simulink model "bh_proto_swingup_OUT_OF_PHASE_CONTROL"  (R2017a)
settings: Solver=ode45  StartTime=0.0  StopTime=22  FixedStep=0.001  RelTol=1e-5  EnableMultiTasking=on
values from neighbouring files (symbols this model uses):
  b3_damp = res_T.b3_damp    [bh_pend_solve_ODE_sys.m]
  Io3_xx = res_T.Io3_xx    [bh_pend_solve_ODE_sys.m]
  L3y = res_T.L3y    [bh_pend_solve_ODE_sys.m]    (also in bh_pend_solve_ODE_sys_custom.m)
  m = res_T.mass3    [bh_pend_solve_ODE_sys_custom.m]
  mass3 = res_T.mass3    [bh_pend_solve_ODE_sys.m]    (also in bh_pend_solve_ODE_sys_custom.m)
  N = 1 + N_steps    [bh_pend_solve_ODE_sys_custom.m]
undefined symbols (not defined in the file or in its folder): L3x, L3z, X, Y, Z
libraries: sm_lib x12, simulink_extras x11, nesl_utility x8, simulink x1
settings Model: Creator=bhorton  LastModifiedBy=bhorton
settings SolverCC: ZeroCrossAlgorithm=Adaptive
settings OptimizationCC: LifeSpan=inf
settings DebuggingCC: SFUnexpectedBacktrackingDiag=warning  SFNoUnconditionalDefaultTransitionDiag=warning  SFExecutionAtInitializationDiag=none
settings GRTTargetCC: TargetLangStandard=C89/C90 (ANSI)
settings ConfigComp: CovMetricSettings=dw  CovHtmlReporting=on  CovSaveCumulativeToWorkspaceVar=on  CovSaveSingleToWorkspaceVar=on  CovExternalEMLEnable=off
settings SimscapeCC: SimscapeLogDataHistory=10000  SelectedTab=Simscape Multibody
settings ExplorerConfigSet: InternalSimMechanicsExplorerSettings="<ExplorerConfiguration><canonicalview>default</canonicalview><AnimationSetting><BasePlaybackSpeed>1.0</BasePlaybackSpeed><PlaybackSpeedFactor>1.0</PlaybackSpeedFactor></AnimationSetting><TilePanel><TileInfo><Tiles Columns=\"1\" Count=\"1\" Rows=\"1\"><Column Left=\"2\" Weight=\"1\"/><Column Left=\"1585\" Weight=\"0.5\"/><Row Top=\"2\" Weight=\"1\"/><Row Top=\"911\" Weight=\"0.5005\"/><Tile Height=\"1\" Width=\"1\" X=\"0\" Y=\"0\"/></Tiles></TileInfo><SceneInfo><SceneViewer><BGColor><R>0.60000002384185791</R><G>0.60000002384185791</G><B>0.60000002384185791</B></BGColor><Camera><DoPerspective>off</DoPerspective><Position><X>0.97226610796774449</X><Y>0.24871023220719646</Y><Z>0.19848014681163439</Z></Position><Center><X>-1.1885447515069814e-08</X><Y>0.12499999495795672</Y><Z>-1.7810067587387124e-09</Z></Center><Up><X>-0.2183009159559649</X><Y>0.17550270816811642</Y><Z>0.9599705774233106</Z></Up><ViewLimDist>1</ViewLimDist><YLim>0.073618170266836078</YLim><XLim>0.12874999999999998</XLim></Camera></SceneViewer></SceneInfo></TilePanel><MechEditorPanel><Cameras/><GfxPanelCameraMap/><VideoCreator><PlaybackSpeedRatio>1.0</PlaybackSpeedRatio><FrameRate>30</FrameRate><VideoFormat>Motion JPEG AVI</VideoFormat><FrameSize>auto</FrameSize></VideoCreator></MechEditorPanel></ExplorerConfiguration>"

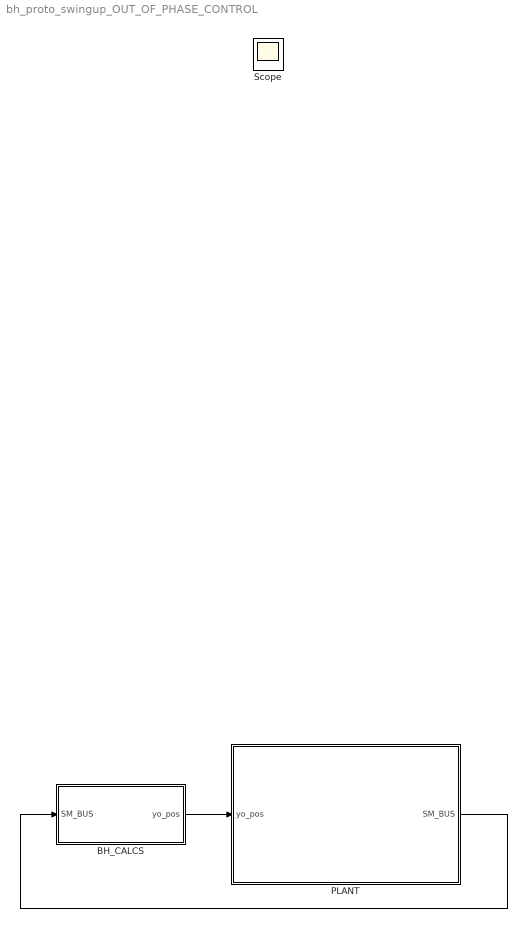
== system bh_proto_swingup_OUT_OF_PHASE_CONTROL ==
  BH_CALCS : Subsystem
  PLANT : Subsystem
  Scope : Scope
  wires:
  PLANT/1(SM_BUS) -> BH_CALCS/1(SM_BUS)
  BH_CALCS/1(yo_pos) -> PLANT/1(yo_pos)

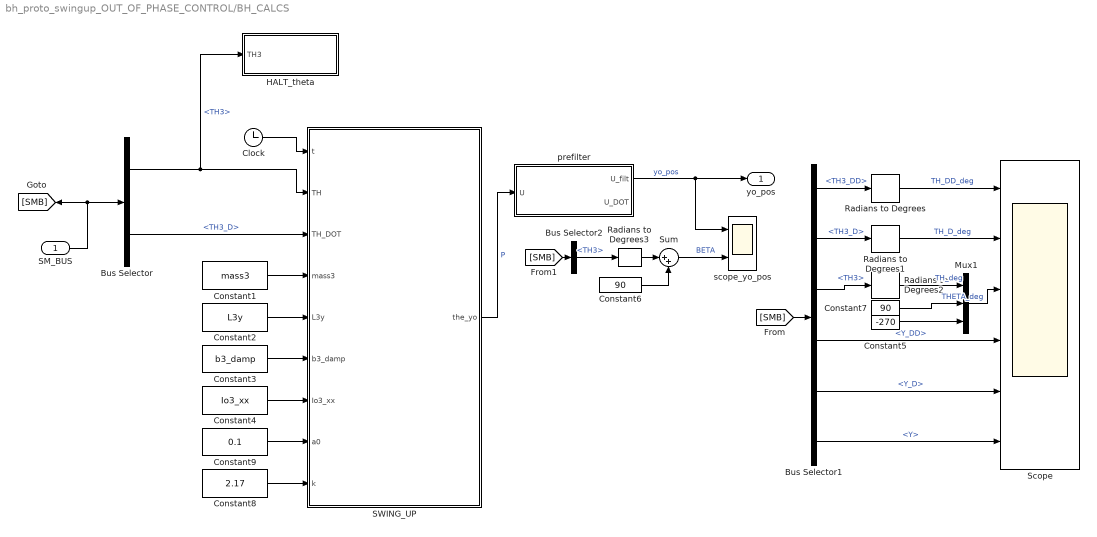
== system bh_proto_swingup_OUT_OF_PHASE_CONTROL/BH_CALCS ==
  SM_BUS : Inport
  Bus Selector : BusSelector  OutputSignals=TH3,TH3_D
  Bus Selector1 : BusSelector  OutputSignals=TH3_DD,TH3_D,TH3,Y_DD,Y_D,Y
  Bus Selector2 : BusSelector  OutputSignals=TH3
  Clock : Clock
  Constant1 : Constant  Value=mass3
  Constant2 : Constant  Value=L3y
  Constant3 : Constant  Value=b3_damp
  Constant4 : Constant  Value=Io3_xx
  Constant5 : Constant  Value=-270
  Constant6 : Constant  Value=90
  Constant7 : Constant  Value=90
  Constant8 : Constant  Value=2.17
  Constant9 : Constant  Value=0.1
  HALT_theta : Subsystem
  Mux1 : Mux  Inputs=3
  Radians to Degrees{,1..3} (4 alike) : simulink_extras/Transformations/Radians to Degrees
  SWING_UP : MATLAB Function  TreatAsAtomicUnit=on  SystemSampleTime=0.001
  Scope : Scope  NumInputPorts=6
  Sum : Sum  Inputs=|++
  prefilter : Subsystem  mask(Derivative Estimation){wn=2*pi*50, p=1}
      mask prompts: wn "Natural frequency, wn (rad/sec)"; p "Damping ratio, p"
      mask help:
      | A simple derivative estimator using a 2nd order representation between input and output.
      |
      | The integrators use a discrete FORWARd Euler rule, and a sample time needs to be specified.
      mask init:
      | str1 = sprintf('wn = %.2f', wn);
      | str2 = sprintf('p  = %.2f', p);
      | %str3 = sprintf('dt = %.2f', dt);
      | %str = char(str1,str2,str3);
      | %str3 = sprintf('dt = %.2f', dt);
      | str = char(str1,str2);
      mask Display: disp(str)
  scope_yo_pos : Scope  NumInputPorts=2
  yo_pos : Outport
  wires:
  prefilter/1(U_filt) -> scope_yo_pos/1, yo_pos/1  "yo_pos"
  SM_BUS/1 -> [SMB], Bus Selector/1
  Bus Selector/1 -> SWING_UP/2(TH), HALT_theta/1(TH3)  "<TH3>"
  Bus Selector/2 -> SWING_UP/3(TH_DOT)  "<TH3_D>"
  Constant3/1 -> SWING_UP/6(b3_damp)
  Constant2/1 -> SWING_UP/5(L3y)
  Constant1/1 -> SWING_UP/4(mass3)
  [SMB] -> Bus Selector1/1
  Bus Selector1/1 -> Radians to Degrees/1  "<TH3_DD>"
  Bus Selector1/2 -> Radians to Degrees1/1  "<TH3_D>"
  Bus Selector1/3 -> Radians to Degrees2/1  "<TH3>"
  Radians to Degrees/1 -> Scope/1  "TH_DD_deg"
  Radians to Degrees1/1 -> Scope/2  "TH_D_deg"
  Radians to Degrees2/1 -> Mux1/1  "TH_deg"
  Bus Selector1/4 -> Scope/4  "<Y_DD>"
  Bus Selector1/5 -> Scope/5  "<Y_D>"
  Bus Selector1/6 -> Scope/6  "<Y>"
  Clock/1 -> SWING_UP/1(t)
  Constant4/1 -> SWING_UP/7(Io3_xx)
  Constant7/1 -> Mux1/2
  Constant9/1 -> SWING_UP/8(a0)
  Constant8/1 -> SWING_UP/9(k)
  Mux1/1 -> Scope/3  "THETA_deg"
  Constant5/1 -> Mux1/3
  SWING_UP/1(the_yo) -> prefilter/1(U)  "P"
  [SMB] -> Bus Selector2/1
  Sum/1 -> scope_yo_pos/2  "BETA"
  Bus Selector2/1 -> Radians to Degrees3/1  "<TH3>"
  Radians to Degrees3/1 -> Sum/1
  Constant6/1 -> Sum/2

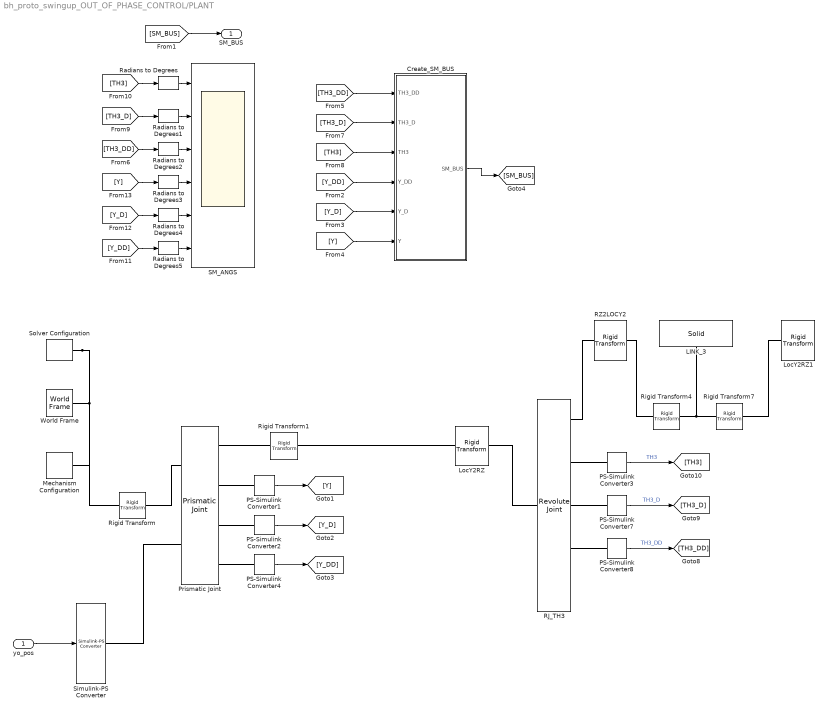
== system bh_proto_swingup_OUT_OF_PHASE_CONTROL/PLANT ==
  yo_pos : Inport
  Create_SM_BUS : Subsystem
  LINK_3 : sm_lib/Body Elements/Solid  InertiaType=CalculateFromGeometry  Mass=1  MassUnits=kg  CenterOfMass=[0 0 0]  CenterOfMassUnits=m  MomentsOfInertia=[1 1 1]  MomentsOfInertiaUnits=kg*m^2  ProductsOfInertia=[0 0 0]  ProductsOfInertiaUnits=kg*m^2  DensityBased=on  Density=density  DensityUnits=kg/(m^3)  DoExposeReferenceFrame=on  SerializedFrames=<Frames/>  GraphicType=FromGeometry  MarkerShape=Sphere  MarkerSize=10  GraphicVisPropType=SimpleVisualProperties  GraphicDiffuseColor=[1.0 0.8 0.4]  GraphicSpecularColor=[0.5 0.5 0.5 1.0]  GraphicAmbientColor=[0.15 0.15 0.15 1.0]  GraphicEmissiveColor=[0.0 0.0 0.0 1.0]  GraphicShininess=75  GraphicOpacity=1.0  GeometryShape=Brick  RectangleSize=[1 1]  RectangleSizeUnits=m  BrickDimensions=[L3x, L3y, L3z ]  BrickDimensionUnits=m  CylinderRadius=1  CylinderRadiusUnits=m  CylinderLength=1  CylinderLengthUnits=m  SphereRadius=1  SphereRadiusUnits=m  EllipsoidRadii=[1 1 1]  EllipsoidRadiiUnits=m  ExtrusionCrossSection=[1 1; -1 1; -1 -1; 1 -1]  ExtrusionCrossSectionUnits=m  ExtrusionLength=1  ExtrusionLengthUnits=m  PolygonNumSides=3  PolygonOuterRadius=1  PolygonOuterRadiusUnits=m  ExtGeomFileType=STEP  ExtGeomFileUnits=m  RevolutionCrossSection=[1 1; 1 -1; 2 -1; 2 1]  RevolutionCrossSectionUnits=m  RevolutionExtent=Full  RevolutionAngle=180  RevolutionAngleUnits=deg
  LocY2RZ : sm_lib/Frames and Transforms/Rigid Transform  TranslationMethod=None  TranslationStandardOffset=0  TranslationLengthUnit=m  TranslationStandardAxis=+Z  TranslationCartesianOffset=[0 0 0]  TranslationROffset=0  TranslationROffsetUnits=m  TranslationZOffset=0  TranslationZOffsetUnits=m  TranslationThetaOffset=0  TranslationThetaOffsetUnits=deg  RotationMethod=AlignedAxes  RotationAngleUnits=deg  RotationStandardAxis=+Z  RotationAngle=0.0  RotationArbitraryAxis=[0 0 1]  FollAlignAxisA=+X  BaseAlignAxisA=+Y  FollAlignAxisB=+Y  BaseAlignAxisB=+Z  RotationSequenceAxes=FollowerAxes  RotationSequence=XYX  RotationSequenceAngles=[0 0 0]  RotationSequenceAnglesUnits=deg  RotationMatrix=[1 0 0; 0 1 0; 0 0 1]
  LocY2RZ1 : sm_lib/Frames and Transforms/Rigid Transform  TranslationMethod=None  TranslationStandardOffset=0  TranslationLengthUnit=m  TranslationStandardAxis=+Z  TranslationCartesianOffset=[0 0 0]  TranslationROffset=0  TranslationROffsetUnits=m  TranslationZOffset=0  TranslationZOffsetUnits=m  TranslationThetaOffset=0  TranslationThetaOffsetUnits=deg  RotationMethod=AlignedAxes  RotationAngleUnits=deg  RotationStandardAxis=+Z  RotationAngle=0.0  RotationArbitraryAxis=[0 0 1]  FollAlignAxisA=+X  BaseAlignAxisA=+Y  FollAlignAxisB=+Y  BaseAlignAxisB=+Z  RotationSequenceAxes=FollowerAxes  RotationSequence=XYX  RotationSequenceAngles=[0 0 0]  RotationSequenceAnglesUnits=deg  RotationMatrix=[1 0 0; 0 1 0; 0 0 1]
  Mechanism Configuration : sm_lib/Utilities/Mechanism Configuration  UniformGravity=Constant  GravityVector=[0 0 -9.80665 ]  GravityUnits=m/s^2  LinearizationDelta=1e-4
  PS-Simulink Converter1 : nesl_utility/PS-Simulink Converter  PhysicalDomain=network_engine_domain  SubClassName=ps_output  LeftPortType=input  RightPortType=output  PseudoPeriodic=off  Frequencies=[]  Unit=m  AffineConversion=off
  PS-Simulink Converter2 : nesl_utility/PS-Simulink Converter  PhysicalDomain=network_engine_domain  SubClassName=ps_output  LeftPortType=input  RightPortType=output  PseudoPeriodic=off  Frequencies=[]  Unit=m/s  AffineConversion=off
  PS-Simulink Converter3 : nesl_utility/PS-Simulink Converter  PhysicalDomain=network_engine_domain  SubClassName=ps_output  LeftPortType=input  RightPortType=output  PseudoPeriodic=off  Frequencies=[]  Unit=rad  AffineConversion=off
  PS-Simulink Converter4 : nesl_utility/PS-Simulink Converter  PhysicalDomain=network_engine_domain  SubClassName=ps_output  LeftPortType=input  RightPortType=output  PseudoPeriodic=off  Frequencies=[]  Unit=m/s^2  AffineConversion=off
  PS-Simulink Converter7 : nesl_utility/PS-Simulink Converter  PhysicalDomain=network_engine_domain  SubClassName=ps_output  LeftPortType=input  RightPortType=output  PseudoPeriodic=off  Frequencies=[]  Unit=rad/s  AffineConversion=off
  PS-Simulink Converter8 : nesl_utility/PS-Simulink Converter  PhysicalDomain=network_engine_domain  SubClassName=ps_output  LeftPortType=input  RightPortType=output  PseudoPeriodic=off  Frequencies=[]  Unit=rad/s^2  AffineConversion=off
  Prismatic Joint : sm_lib/Joints/Prismatic Joint  SenseConstraintForce=off  SenseConstraintForceX=off  SenseConstraintForceY=off  SenseConstraintForceZ=off  SenseConstraintTorque=off  SenseConstraintTorqueX=off  SenseConstraintTorqueY=off  SenseConstraintTorqueZ=off  SenseTotalForce=off  SenseTotalForceX=off  SenseTotalForceY=off  SenseTotalForceZ=off  SenseTotalTorque=off  SenseTotalTorqueX=off  SenseTotalTorqueY=off  SenseTotalTorqueZ=off  CompositeWrenchDir=FollowerOnBase  CompositeWrenchFrame=BaseFrame  EquilibriumPosition=0  EquilibriumPositionUnits=m  SpringStiffness=0  SpringStiffnessUnits=N/m  DampingCoefficient=0  DampingCoefficientUnits=N/(m/s)  TorqueActuationMode=ComputedTorque  MotionActuationMode=InputMotion  SensePosition=on  SenseVelocity=on  SenseAcceleration=on  SenseTorqueForce=off  PositionTargetSpecify=off  PositionTargetPriority=High  PositionTargetValue=0  PositionTargetValueUnits=m  VelocityTargetSpecify=off  VelocityTargetPriority=High  VelocityTargetValue=0  VelocityTargetValueUnits=m/s
  RJ_TH3 : sm_lib/Joints/Revolute Joint  SenseConstraintForce=on  SenseConstraintForceX=off  SenseConstraintForceY=off  SenseConstraintForceZ=off  SenseConstraintTorque=off  SenseConstraintTorqueX=off  SenseConstraintTorqueY=off  SenseConstraintTorqueZ=off  SenseTotalForce=off  SenseTotalForceX=off  SenseTotalForceY=off  SenseTotalForceZ=off  SenseTotalTorque=off  SenseTotalTorqueX=off  SenseTotalTorqueY=off  SenseTotalTorqueZ=off  CompositeWrenchDir=BaseOnFollower  CompositeWrenchFrame=BaseFrame  EquilibriumPosition=0  EquilibriumPositionUnits=deg  SpringStiffness=0  SpringStiffnessUnits=N*m/deg  DampingCoefficient=b3_damp  DampingCoefficientUnits=N*m/(rad/s)  TorqueActuationMode=NoTorque  MotionActuationMode=ComputedMotion  SensePosition=on  SenseVelocity=on  SenseAcceleration=on  SenseTorqueForce=off  PositionTargetSpecify=on  PositionTargetPriority=Low  PositionTargetValue=-90  PositionTargetValueUnits=deg  VelocityTargetSpecify=on  VelocityTargetPriority=High  VelocityTargetValue=0  VelocityTargetValueUnits=rad/s
      settings: AttributesFormatString=|
      | %<DampingCoefficient>
      | %<PositionTargetValue>
      | %<VelocityTargetValue>
  RZ2LOCY2 : sm_lib/Frames and Transforms/Rigid Transform  TranslationMethod=None  TranslationStandardOffset=0  TranslationLengthUnit=m  TranslationStandardAxis=+Z  TranslationCartesianOffset=[0 0 0]  TranslationROffset=0  TranslationROffsetUnits=m  TranslationZOffset=0  TranslationZOffsetUnits=m  TranslationThetaOffset=0  TranslationThetaOffsetUnits=deg  RotationMethod=AlignedAxes  RotationAngleUnits=deg  RotationStandardAxis=+Z  RotationAngle=0.0  RotationArbitraryAxis=[0 0 1]  FollAlignAxisA=+Y  BaseAlignAxisA=+X  FollAlignAxisB=+X  BaseAlignAxisB=+Z  RotationSequenceAxes=FollowerAxes  RotationSequence=XYX  RotationSequenceAngles=[0 0 0]  RotationSequenceAnglesUnits=deg  RotationMatrix=[1 0 0; 0 1 0; 0 0 1]
  Radians to Degrees{,1..5} (6 alike) : simulink_extras/Transformations/Radians to Degrees
  Rigid Transform : sm_lib/Frames and Transforms/Rigid Transform  TranslationMethod=None  TranslationStandardOffset=0  TranslationLengthUnit=m  TranslationStandardAxis=+Z  TranslationCartesianOffset=[0 0 0]  TranslationROffset=0  TranslationROffsetUnits=m  TranslationZOffset=0  TranslationZOffsetUnits=m  TranslationThetaOffset=0  TranslationThetaOffsetUnits=deg  RotationMethod=AlignedAxes  RotationAngleUnits=deg  RotationStandardAxis=+Z  RotationAngle=0.0  RotationArbitraryAxis=[0 0 1]  FollAlignAxisA=+X  BaseAlignAxisA=+X  FollAlignAxisB=+Z  BaseAlignAxisB=+Y  RotationSequenceAxes=FollowerAxes  RotationSequence=XYX  RotationSequenceAngles=[0 0 0]  RotationSequenceAnglesUnits=deg  RotationMatrix=[1 0 0; 0 1 0; 0 0 1]
  Rigid Transform1 : sm_lib/Frames and Transforms/Rigid Transform  TranslationMethod=None  TranslationStandardOffset=0  TranslationLengthUnit=m  TranslationStandardAxis=+Z  TranslationCartesianOffset=[0 0 0]  TranslationROffset=0  TranslationROffsetUnits=m  TranslationZOffset=0  TranslationZOffsetUnits=m  TranslationThetaOffset=0  TranslationThetaOffsetUnits=deg  RotationMethod=AlignedAxes  RotationAngleUnits=deg  RotationStandardAxis=+Z  RotationAngle=0.0  RotationArbitraryAxis=[0 0 1]  FollAlignAxisA=+X  BaseAlignAxisA=+X  FollAlignAxisB=+Y  BaseAlignAxisB=+Z  RotationSequenceAxes=FollowerAxes  RotationSequence=XYX  RotationSequenceAngles=[0 0 0]  RotationSequenceAnglesUnits=deg  RotationMatrix=[1 0 0; 0 1 0; 0 0 1]
  Rigid Transform4 : sm_lib/Frames and Transforms/Rigid Transform  TranslationMethod=StandardAxis  TranslationStandardOffset=L3y/2  TranslationLengthUnit=m  TranslationStandardAxis=+Y  TranslationCartesianOffset=[0 0 0]  TranslationROffset=0  TranslationROffsetUnits=m  TranslationZOffset=0  TranslationZOffsetUnits=m  TranslationThetaOffset=0  TranslationThetaOffsetUnits=deg  RotationMethod=None  RotationAngleUnits=deg  RotationStandardAxis=+Z  RotationAngle=0.0  RotationArbitraryAxis=[0 0 1]  FollAlignAxisA=+X  BaseAlignAxisA=+Y  FollAlignAxisB=+Y  BaseAlignAxisB=+Z  RotationSequenceAxes=FollowerAxes  RotationSequence=XYX  RotationSequenceAngles=[0 0 0]  RotationSequenceAnglesUnits=deg  RotationMatrix=[1 0 0; 0 1 0; 0 0 1]
  Rigid Transform7 : sm_lib/Frames and Transforms/Rigid Transform  TranslationMethod=StandardAxis  TranslationStandardOffset=L3y/2  TranslationLengthUnit=m  TranslationStandardAxis=+Y  TranslationCartesianOffset=[0 0 0]  TranslationROffset=0  TranslationROffsetUnits=m  TranslationZOffset=0  TranslationZOffsetUnits=m  TranslationThetaOffset=0  TranslationThetaOffsetUnits=deg  RotationMethod=None  RotationAngleUnits=deg  RotationStandardAxis=+Z  RotationAngle=0.0  RotationArbitraryAxis=[0 0 1]  FollAlignAxisA=+X  BaseAlignAxisA=+Y  FollAlignAxisB=+Y  BaseAlignAxisB=+Z  RotationSequenceAxes=FollowerAxes  RotationSequence=XYX  RotationSequenceAngles=[0 0 0]  RotationSequenceAnglesUnits=deg  RotationMatrix=[1 0 0; 0 1 0; 0 0 1]
  SM_ANGS : Scope  NumInputPorts=6
  Simulink-PS Converter : nesl_utility/Simulink-PS Converter  PhysicalDomain=network_engine_domain  SubClassName=ps_input  LeftPortType=input  RightPortType=output  PseudoPeriodic=off  Frequencies=[]  NoiseDistribution=none  NoiseParameters=[]  Unit=m  AffineConversion=off  FilteringAndDerivatives=filter  SimscapeFilterOrder=2  InputFilterTimeConstant=0.01  UdotUserProvided=2
  Solver Configuration : nesl_utility/Solver Configuration  PhysicalDomain=network_engine_domain  SubClassName=solver  LeftPortType=input  RightPortType=generic  Accelerate=off  Tones=[]  Harmonics=[]  SimulateNoise=off  Profile=off  UseLocalSampling=off  EnableSwitchedLinearOptims=on  FrequencyDomain=off  UseCCode=off  RelTol=0.001  AbsTol=1e-06  MinStep=1e-09  ToWorkspace=off  RevertToSquareIcSolve=off  NumHomotopyIterations=100  PhasorMode=off  PhasorModeNumHarmonics=1  OverrideAbsTol=off  DoDC=off  ResidualTolerance=1e-09  UseLocalSolver=off  LocalSolverChoice=NE_TRAPEZOIDAL_ADVANCER  LocalSolverSampleTime=0.01  DoFixedCost=off  MaxNonlinIter=3  MaxModeIter=2  LinearAlgebra=Sparse  DelaysMemoryBudget=1024  AutomaticFiltering=off  FilteringTimeConstant=0.001
  World Frame : sm_lib/Frames and Transforms/World Frame
  SM_BUS : Outport
  wires:
  [TH3] -> Create_SM_BUS/3(TH3)
  [Y] -> Radians to Degrees3/1
  [Y] -> Create_SM_BUS/6(Y)
  PS-Simulink Converter7/1 -> [TH3_D]  "TH3_D"
  yo_pos/1 -> Simulink-PS Converter/1
  [TH3_D] -> Radians to Degrees1/1
  Create_SM_BUS/1(SM_BUS) -> [SM_BUS]
  [TH3_D] -> Create_SM_BUS/2(TH3_D)
  [TH3_DD] -> Create_SM_BUS/1(TH3_DD)
  PS-Simulink Converter3/1 -> [TH3]  "TH3"
  PS-Simulink Converter1/1 -> [Y]
  [SM_BUS] -> SM_BUS/1
  [TH3] -> Radians to Degrees/1
  PS-Simulink Converter8/1 -> [TH3_DD]  "TH3_DD"
  PS-Simulink Converter4/1 -> [Y_DD]
  [Y_DD] -> Create_SM_BUS/4(Y_DD)
  PS-Simulink Converter2/1 -> [Y_D]
  [Y_DD] -> Radians to Degrees5/1
  [TH3_DD] -> Radians to Degrees2/1
  [Y_D] -> Create_SM_BUS/5(Y_D)
  [Y_D] -> Radians to Degrees4/1
  Radians to Degrees/1 -> SM_ANGS/1
  Radians to Degrees1/1 -> SM_ANGS/2
  Radians to Degrees2/1 -> SM_ANGS/3
  Radians to Degrees3/1 -> SM_ANGS/4
  Radians to Degrees4/1 -> SM_ANGS/5
  Radians to Degrees5/1 -> SM_ANGS/6
  connections:
  Solver Configuration/RConn1 -- World Frame/RConn1 -- Rigid Transform/LConn1 -- Mechanism Configuration/RConn1
  RZ2LOCY2/RConn1 -- Rigid Transform4/LConn1
  PS-Simulink Converter3/LConn1 -- RJ_TH3/RConn2
  Prismatic Joint/LConn1 -- Rigid Transform/RConn1
  PS-Simulink Converter4/LConn1 -- Prismatic Joint/RConn4
  LocY2RZ1/LConn1 -- Rigid Transform7/RConn1
  Prismatic Joint/RConn2 -- PS-Simulink Converter1/LConn1
  LocY2RZ/LConn1 -- Rigid Transform1/RConn1
  RJ_TH3/LConn1 -- LocY2RZ/RConn1
  Simulink-PS Converter/RConn1 -- Prismatic Joint/LConn2
  Rigid Transform4/RConn1 -- LINK_3/RConn1 -- Rigid Transform7/LConn1
  RJ_TH3/RConn3 -- PS-Simulink Converter7/LConn1
  Rigid Transform1/LConn1 -- Prismatic Joint/RConn1
  RJ_TH3/RConn4 -- PS-Simulink Converter8/LConn1
  PS-Simulink Converter2/LConn1 -- Prismatic Joint/RConn3
  RZ2LOCY2/LConn1 -- RJ_TH3/RConn1

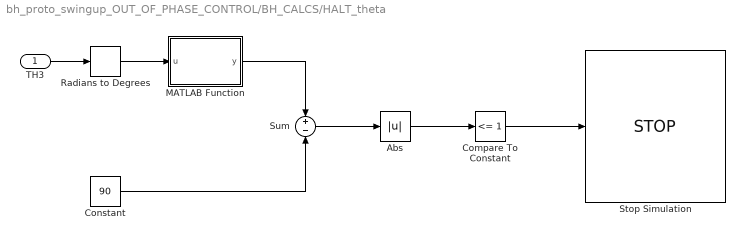
== system bh_proto_swingup_OUT_OF_PHASE_CONTROL/BH_CALCS/HALT_theta ==
  TH3 : Inport
  Abs : Abs
  Compare To Constant : simulink/Logic and Bit Operations/Compare To Constant  relop=<=  const=1  OutDataTypeStr=boolean
  Constant : Constant  Value=90
  MATLAB Function : MATLAB Function  TreatAsAtomicUnit=on
  Radians to Degrees : simulink_extras/Transformations/Radians to Degrees
  Stop Simulation : Stop
  Sum : Sum  Inputs=+|-
  wires:
  TH3/1 -> Radians to Degrees/1
  Radians to Degrees/1 -> MATLAB Function/1(u)
  Constant/1 -> Sum/2
  Sum/1 -> Abs/1
  Abs/1 -> Compare To Constant/1
  Compare To Constant/1 -> Stop Simulation/1
  MATLAB Function/1(y) -> Sum/1

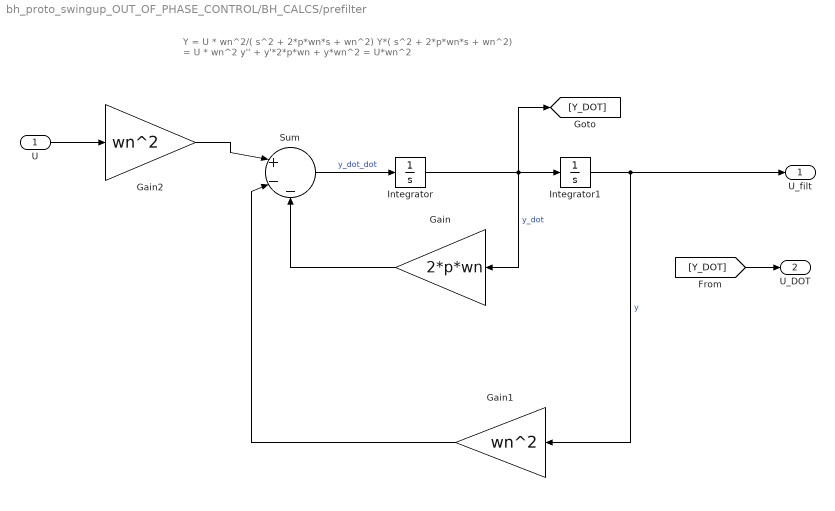
== system bh_proto_swingup_OUT_OF_PHASE_CONTROL/BH_CALCS/prefilter ==
  note: Y = U *     wn^2/( s^2 + 2*p*wn*s + wn^2)
      | Y*( s^2 + 2*p*wn*s + wn^2) = U * wn^2
      |
      | y'' + y'*2*p*wn + y*wn^2 = U*wn^2
  U : Inport
  Gain : Gain  Gain=2*p*wn
  Gain1 : Gain  Gain=wn^2
  Gain2 : Gain  Gain=wn^2
  Integrator : Integrator
  Integrator1 : Integrator
  Sum : Sum  Inputs=|+--
  U_filt : Outport
  U_DOT : Outport  Port=2
  wires:
  Integrator/1 -> Integrator1/1, [Y_DOT], Gain/1  "y_dot"
  Sum/1 -> Integrator/1  "y_dot_dot"
  Integrator1/1 -> Gain1/1, U_filt/1  "y"
  U/1 -> Gain2/1
  Gain2/1 -> Sum/1
  Gain/1 -> Sum/3
  Gain1/1 -> Sum/2
  [Y_DOT] -> U_DOT/1

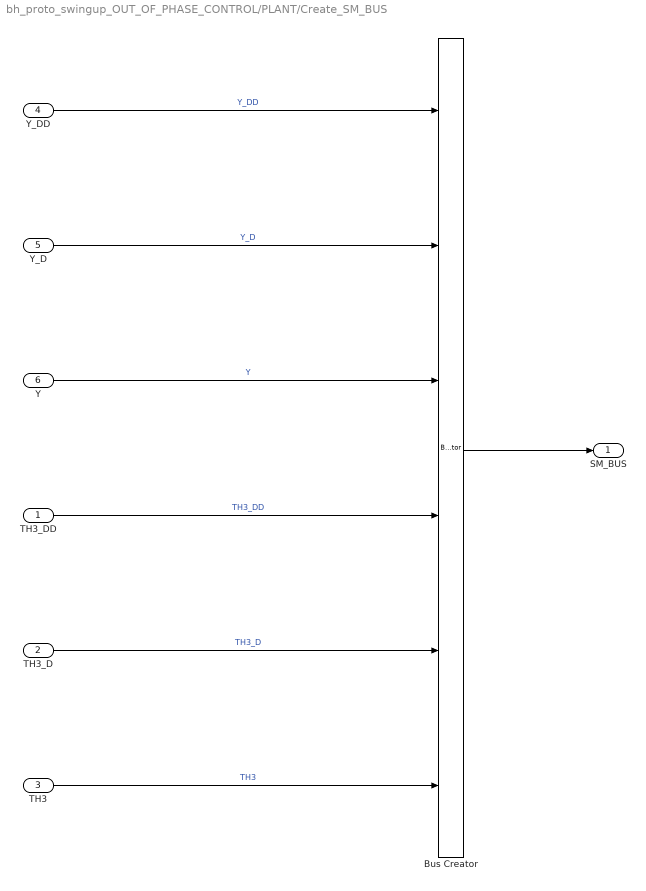
== system bh_proto_swingup_OUT_OF_PHASE_CONTROL/PLANT/Create_SM_BUS ==
  TH3_DD : Inport
  TH3_D : Inport  Port=2
  TH3 : Inport  Port=3
  Y_DD : Inport  Port=4
  Y_D : Inport  Port=5
  Y : Inport  Port=6
  Bus Creator : BusCreator  Inputs=6
  SM_BUS : Outport
  wires:
  Bus Creator/1 -> SM_BUS/1
  TH3/1 -> Bus Creator/6  "TH3"
  TH3_D/1 -> Bus Creator/5  "TH3_D"
  TH3_DD/1 -> Bus Creator/4  "TH3_DD"
  Y_D/1 -> Bus Creator/2  "Y_D"
  Y/1 -> Bus Creator/3  "Y"
  Y_DD/1 -> Bus Creator/1  "Y_DD"

== matlab function bh_proto_swingup_OUT_OF_PHASE_CONTROL/BH_CALCS/HALT_theta/MATLAB Function ==
  data: u input; y output
function y = fcn(u)
coder.extrinsic('wrapTo180');
y = 0;
y = wrapTo180(u);

== matlab function bh_proto_swingup_OUT_OF_PHASE_CONTROL/BH_CALCS/SWING_UP ==
  data: t input; TH input; the_yo output; TH_DOT input; mass3 input; L3y input; b3_damp input; Io3_xx input; a0 input; k input
function the_yo    = fcn(t, TH, TH_DOT, mass3, L3y, b3_damp, Io3_xx, a0, k)

persistent last_yo 
persistent tf_is_doing_phase_1
persistent last_theta_dot
persistent t_at_end_phase_1
persistent t_start

if( isempty(last_yo) )
    last_yo             = 0;
    tf_is_doing_phase_1 = true;
    last_theta_dot      = 0;
    t_at_end_phase_1    = 0;
    t_start             = t;
end

my_t          = t - t_start;
the_yo        = 0;
    theta     = TH;   
    theta_dot = TH_DOT;

BETA          = theta + pi/2;
wn            = sqrt(mass3*9.81*L3y/Io3_xx); 
T             = 1/(wn/(2*pi));

% h             =   0.5 * L3y * sin(theta);  
% E_goal        = mass3 * 9.81 *  (L3y/2);
% PE            = mass3 * 9.81 * h;
% KE            = 0.5 * Io3_xx * (theta_dot^2);
% E             = PE;   %E     = PE + KE;
% E_diff        = E - E_goal;

phi           = atan2( -1*theta_dot/wn, BETA);

if(my_t<=3*T)
    the_yo         = a0 * sin(  1.0*my_t*wn );
    last_yo        = the_yo;
    last_theta_dot = theta_dot;
    return
end


if(tf_is_doing_phase_1==true)

    if(sign(theta_dot) ~= sign(last_theta_dot) )
        tf_is_doing_phase_1 = false;
        t_at_end_phase_1    = my_t;
    end
        
    return
end

% specify the yo_pos
Y2        = a0 * sin(k*phi - pi ) ;
the_yo    = Y2;
